simulink model "complex_multiplier_co_sim"  (Simulink 8.0)
settings: Solver=VariableStepDiscrete  StartTime=0.0  StopTime=100  RelTol=1e-3
libraries: xbsIndex_r4 x25
settings Model: Creator=dell  LastModifiedBy=dell

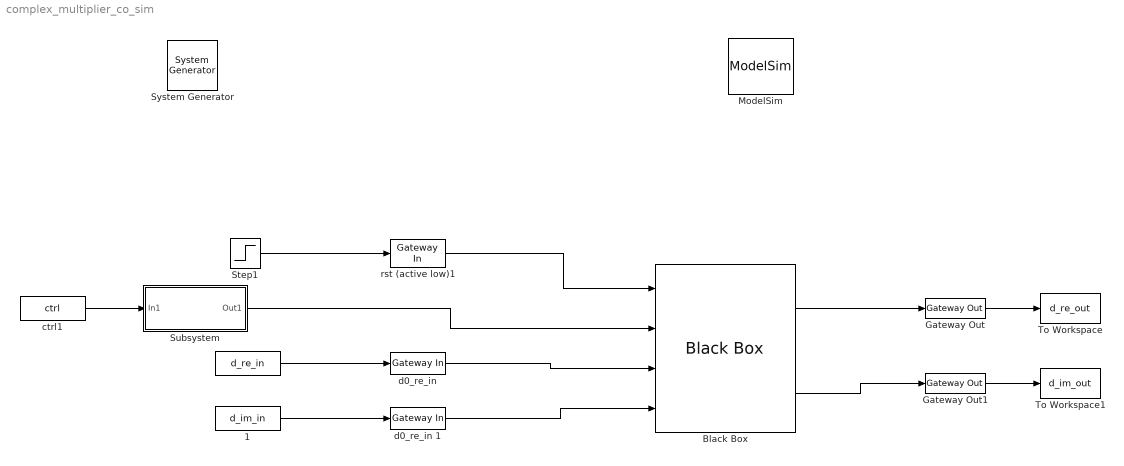
== system complex_multiplier_co_sim ==
  " " : FromWorkspace  VariableName=d_re_in  SampleTime=1  Interpolate=off  OutputAfterFinalValue=Setting to zero
  " 1" : FromWorkspace  VariableName=d_im_in  SampleTime=1  Interpolate=off  OutputAfterFinalValue=Setting to zero
  " System Generator" : xbsIndex_r4/ System Generator  Tag=genX  xilinxfamily=Kintex7  part=xc7k325t  speed=-3  package=fbg676  synthesis_tool=XST  clock_wrapper=Clock Enables  directory=./netlist  proj_type=Project Navigator  Synth_file=XST Defaults  Impl_file=ISE Defaults  testbench=off  simulink_period=1  sysclk_period=10  dcm_input_clock_period=10  incr_netlist=off  trim_vbits=Everywhere in SubSystem  dbl_ovrd=According to Block Masks  core_generation=According to Block Masks  run_coregen=off  deprecated_control=off  eval_field=0  block_type=sysgen
  Black Box : xbsIndex_r4/Black Box  init_code=complex_multiplier_config  sim_method=External co-simulator  engine_block=ModelSim  verbose=off  block_type=blackbox2
  Gateway Out : xbsIndex_r4/Gateway Out  inherit_from_input=off  hdl_port=on  timing_constraint=None  locs_specified=off  LOCs={}  UseAsDAC=off  DACChannel='1'  block_type=gatewayout
  Gateway Out1 : xbsIndex_r4/Gateway Out  inherit_from_input=off  hdl_port=on  timing_constraint=None  locs_specified=off  LOCs={}  UseAsDAC=off  DACChannel='1'  block_type=gatewayout
  ModelSim : xbsIndex_r4/ModelSim  dir=./modelsim  waveform=on  leave_open=on  skip_compile=off  use_unisim=off  use_ver_xilinxcorelib=off  custom_scripts=on  post_vsim_script=./before.do  startup_timeout=40  block_type=hdlcosim
      settings: infoedit="Allow other blocks to schedule HDL co-simulation tasks.<br><br>Note that selecting \"Skip compilation\" when inappropriate can cause simulation errors and failures. Please refer to the block help for details."
  Step1 : Step  SampleTime=1
  Subsystem : Subsystem
  To Workspace : ToWorkspace  VariableName=d_re_out  SampleTime=-1  SaveFormat=Timeseries
  To Workspace1 : ToWorkspace  VariableName=d_im_out  SampleTime=-1  SaveFormat=Timeseries
  ctrl1 : FromWorkspace  VariableName=ctrl  SampleTime=1  Interpolate=off  OutputAfterFinalValue=Setting to zero
  "d0_re_in " : xbsIndex_r4/Gateway In  gui_display_data_type=Boolean  arith_type=Boolean  n_bits=4  bin_pt=0  preci_type=Single  exp_width=8  frac_width=24  quantization="Round  (unbiased: +/- Inf)"  overflow=Saturate  period=1  dbl_ovrd=off  timing_constraint=None  locs_specified=off  LOCs={}  UseAsADC=off  ADCChannel='1'  inherit_from_input=off  hdl_port=on  block_type=gatewayin
      settings: xl_area=[0, 0, 0, 0, 0, 0, 0]  block_version=VER_STRING_GOES_HERE
  d0_re_in 1 : xbsIndex_r4/Gateway In  gui_display_data_type=Boolean  arith_type=Boolean  n_bits=4  bin_pt=0  preci_type=Single  exp_width=8  frac_width=24  quantization="Round  (unbiased: +/- Inf)"  overflow=Saturate  period=1  dbl_ovrd=off  timing_constraint=None  locs_specified=off  LOCs={}  UseAsADC=off  ADCChannel='1'  inherit_from_input=off  hdl_port=on  block_type=gatewayin
      settings: xl_area=[0, 0, 0, 0, 0, 0, 0]  block_version=VER_STRING_GOES_HERE
  rst (active low)1 : xbsIndex_r4/Gateway In  gui_display_data_type=Boolean  arith_type=Boolean  n_bits=10  bin_pt=8  preci_type=Single  exp_width=8  frac_width=24  quantization="Round  (unbiased: +/- Inf)"  overflow=Saturate  period=1  dbl_ovrd=off  timing_constraint=None  locs_specified=off  LOCs={}  UseAsADC=off  ADCChannel='1'  inherit_from_input=off  hdl_port=on  block_type=gatewayin
      settings: xl_area=[0, 0, 0, 0, 0, 0, 0]  block_version=VER_STRING_GOES_HERE
  wires:
  Step1/1 -> rst (active low)1/1
  ctrl1/1 -> Subsystem/1(In1)
  " "/1 -> "d0_re_in "/1
  Subsystem/1(Out1) -> Black Box/2
  rst (active low)1/1 -> Black Box/1
  " 1"/1 -> d0_re_in 1/1
  d0_re_in 1/1 -> Black Box/4
  "d0_re_in "/1 -> Black Box/3
  Gateway Out/1 -> To Workspace/1
  Gateway Out1/1 -> To Workspace1/1
  Black Box/1 -> Gateway Out/1
  Black Box/2 -> Gateway Out1/1

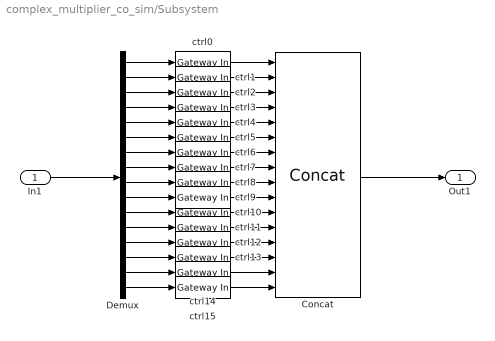
== system complex_multiplier_co_sim/Subsystem ==
  In1 : Inport
  Concat : xbsIndex_r4/Concat  num_inputs=16  dbl_ovrd=off  block_type=concat
  Demux : Demux  Outputs=16
  ctrl{0..15} (16 alike) : xbsIndex_r4/Gateway In  gui_display_data_type=Boolean  arith_type=Boolean  n_bits=16  bin_pt=0  preci_type=Single  exp_width=8  frac_width=24  quantization="Round  (unbiased: +/- Inf)"  overflow=Saturate  period=1  dbl_ovrd=off  timing_constraint=None  locs_specified=off  LOCs={}  UseAsADC=off  ADCChannel='1'  inherit_from_input=off  hdl_port=on  block_type=gatewayin
      settings: xl_area=[0, 0, 0, 0, 0, 0, 0]  block_version=VER_STRING_GOES_HERE
  Out1 : Outport
  wires:
  Demux/1 -> ctrl0/1
  Demux/2 -> ctrl1/1
  Demux/3 -> ctrl2/1
  Demux/12 -> ctrl11/1
  Demux/15 -> ctrl14/1
  Demux/6 -> ctrl5/1
  Demux/11 -> ctrl10/1
  Demux/13 -> ctrl12/1
  Demux/16 -> ctrl15/1
  Demux/10 -> ctrl9/1
  Demux/5 -> ctrl4/1
  Demux/4 -> ctrl3/1
  Demux/14 -> ctrl13/1
  Demux/7 -> ctrl6/1
  Demux/8 -> ctrl7/1
  Demux/9 -> ctrl8/1
  ctrl0/1 -> Concat/1
  ctrl1/1 -> Concat/2
  ctrl2/1 -> Concat/3
  ctrl3/1 -> Concat/4
  ctrl4/1 -> Concat/5
  ctrl5/1 -> Concat/6
  ctrl6/1 -> Concat/7
  ctrl7/1 -> Concat/8
  ctrl8/1 -> Concat/9
  ctrl9/1 -> Concat/10
  ctrl10/1 -> Concat/11
  ctrl11/1 -> Concat/12
  ctrl12/1 -> Concat/13
  ctrl13/1 -> Concat/14
  ctrl14/1 -> Concat/15
  ctrl15/1 -> Concat/16
  In1/1 -> Demux/1
  Concat/1 -> Out1/1
